simulink model "observador"  (R2025a)
settings: Solver=VariableStepAuto  StartTime=0.0  StopTime=10.0  RelTol=1e-3
undefined symbols (not defined in the file): A, b, c, la
settings Model: Creator=sergi  LastModifiedBy=sergi

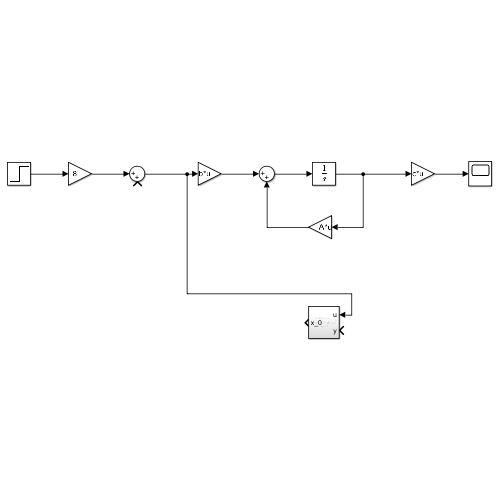
[thumbnail: Simulink's stored preview of the top-level diagram]
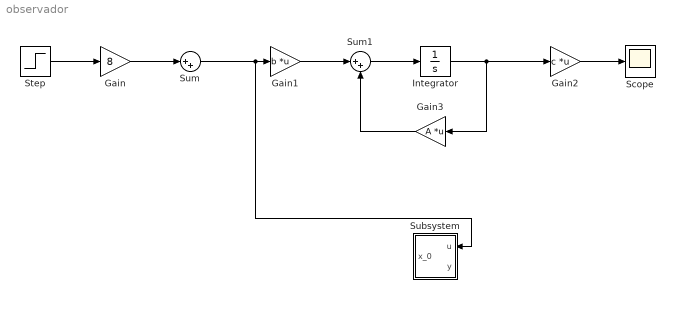
== system observador ==
  Gain : Gain  Gain=8
  Gain1 : Gain  Gain=b  Multiplication=Matrix(K*u)
  Gain2 : Gain  Gain=c  Multiplication=Matrix(K*u)
  Gain3 : Gain  Gain=A  Multiplication=Matrix(K*u)
  Integrator : Integrator
  Scope : Scope
  Step : Step  SampleTime=0
  Subsystem : Subsystem
  Sum : Sum  Inputs=|++
  Sum1 : Sum  Inputs=|++
  wires:
  Step/1 -> Gain/1
  Sum/1 -> Subsystem/1(u), Gain1/1
  Gain1/1 -> Sum1/1
  Integrator/1 -> Gain3/1, Gain2/1
  Sum1/1 -> Integrator/1
  Gain/1 -> Sum/1
  Gain2/1 -> Scope/1
  Gain3/1 -> Sum1/2

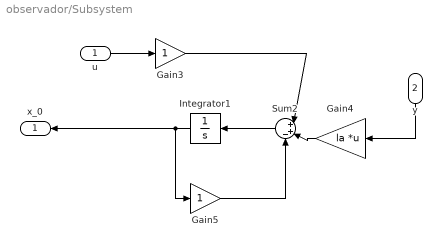
== system observador/Subsystem ==
  u : Inport
  y : Inport  Port=2
  Gain3 : Gain
  Gain4 : Gain  Gain=la  Multiplication=Matrix(K*u)
  Gain5 : Gain
  Integrator1 : Integrator
  Sum2 : Sum  Inputs=|++-
  x_0 : Outport
  wires:
  y/1 -> Gain4/1
  Integrator1/1 -> x_0/1, Gain5/1
  Gain5/1 -> Sum2/3
  Gain4/1 -> Sum2/2
  Gain3/1 -> Sum2/1
  Sum2/1 -> Integrator1/1
  u/1 -> Gain3/1
